simulink model "float_sch_TemplateMatchingContinuous"  (R2020a)
settings: Solver=VariableStepAuto  StartTime=0  StopTime=5  RelTol=1e-3
values from neighbouring files (symbols this model uses):
  buffer_rec = length(template)    [float_sch_run_TemplateMatchingCentered.m]    (also in float_sch_run_TemplateMatchingContinuous.m)
  fs = 30000    [float_sch_run_TemplateMatchingCentered.m]    (also in float_sch_run_TemplateMatchingContinuous.m)
  refractory = 10^-3    (= 0.001)    [float_sch_run_TemplateMatchingCentered.m]    (also in float_sch_run_TemplateMatchingContinuous.m)
  score = [4500]    [float_sch_run_TemplateMatchingCentered.m]    (also in float_sch_run_TemplateMatchingContinuous.m)
  template = double(mean_waveform{1, 1})'    [float_sch_run_TemplateMatchingCentered.m]    (also in float_sch_run_TemplateMatchingContinuous.m)
libraries: dsparch4 x2, simulink x2, dspswit3 x1, hdlsllib x1
settings Model: Creator=sbuccelli  LastModifiedBy=diflo

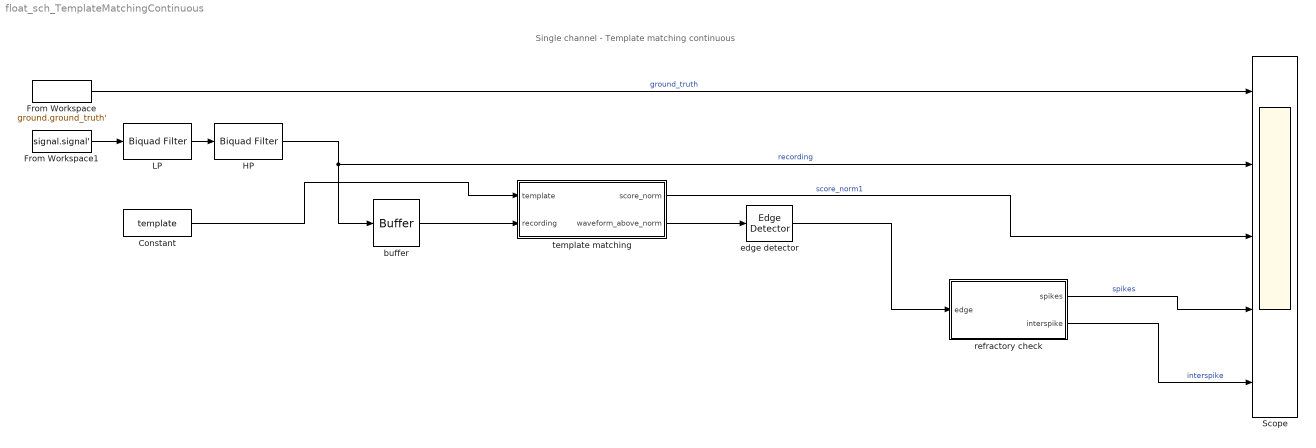
== system float_sch_TemplateMatchingContinuous ==
  note: Single channel - Template matching continuous
  Constant : Constant  Value=template
  From Workspace : FromWorkspace  VariableName=ground.ground_truth'  SampleTime=1/fs
  From Workspace1 : FromWorkspace  VariableName=signal.signal'  SampleTime=1/fs
  HP : dsparch4/Biquad Filter  Tag=BlockMethodSubSystem  FilterSource=Dialog parameters  CoeffSource=Specify via dialog  FilterObject=BQF  IIRFiltStruct=Direct form II  BiQuadCoeffs=[1 -2 1 1 -1.93529438685999167 0.93912079880642374;1 -1 0 1 -0.939062505817492399 0]  ScaleValues=[0.968603796416603768;0.969531252908746199;1]  IC=0  ICnum=0  ICden=0  a0Flag=Warning  optimizeScaleValues=on  ScaleValueMode=Specify via input port (g)  roundingMode=Floor  overflowMode=off  scaleValueFracLength=14  denProdOutputFracLength=30  denAccumFracLength=30  secondMemoryFracLength=15
  LP : dsparch4/Biquad Filter  Tag=BlockMethodSubSystem  FilterSource=Dialog parameters  CoeffSource=Specify via dialog  FilterObject=BQF  IIRFiltStruct=Direct form II  BiQuadCoeffs=[1 1 0 1 -0.509525449494428795 0]  ScaleValues=[0.245237275252785547;1]  IC=0  ICnum=0  ICden=0  a0Flag=Warning  optimizeScaleValues=on  ScaleValueMode=Specify via input port (g)  roundingMode=Floor  overflowMode=off  scaleValueFracLength=14  denProdOutputFracLength=30  denAccumFracLength=30  secondMemoryFracLength=15
  Scope : Scope  NumInputPorts=5
  buffer : Buffer  N=buffer_rec  V=buffer_overlap  OutputFrames=off
  edge detector : dspswit3/Edge Detector  InputProcessing=Columns as channels (frame based)
      settings: SourceProductBaseCode=DS
  refractory check : Subsystem
  template matching : Subsystem
  wires:
  Constant/1 -> template matching/1(template)
  HP/1 -> Scope/2, buffer/1  "recording"
  buffer/1 -> template matching/2(recording)
  From Workspace1/1 -> LP/1
  template matching/2(waveform_above_norm) -> edge detector/1
  From Workspace/1 -> Scope/1  "ground_truth"
  template matching/1(score_norm) -> Scope/3  "score_norm1"
  edge detector/1 -> refractory check/1("  edge")
  refractory check/1(" spikes") -> Scope/4  "spikes"
  refractory check/2(interspike) -> Scope/5  "interspike"
  LP/1 -> HP/1

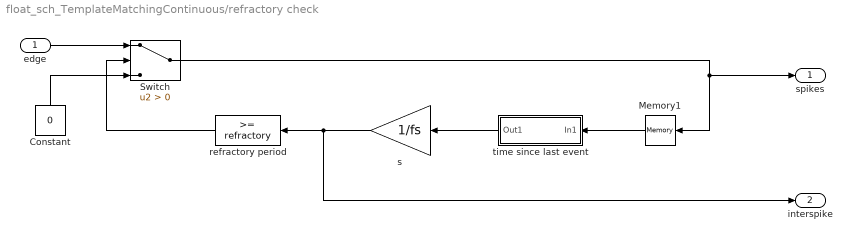
== system float_sch_TemplateMatchingContinuous/refractory check ==
  "  edge" : Inport
  Constant : Constant  Value=0
  Memory1 : Memory  InheritSampleTime=on
  Switch : Switch  Criteria=u2 > Threshold
  refractory period : simulink/Logic and Bit Operations/Compare To Constant  relop=>=  const=refractory  OutDataTypeStr=boolean
  s : Gain  Gain=1/fs  ParamDataTypeStr=double
  time since last event : Subsystem
  " spikes" : Outport
  interspike : Outport  Port=2
  wires:
  "  edge"/1 -> Switch/1
  Memory1/1 -> time since last event/1(In1)
  time since last event/1(Out1) -> s/1
  Constant/1 -> Switch/3
  s/1 -> refractory period/1, interspike/1
  Switch/1 -> " spikes"/1, Memory1/1
  refractory period/1 -> Switch/2

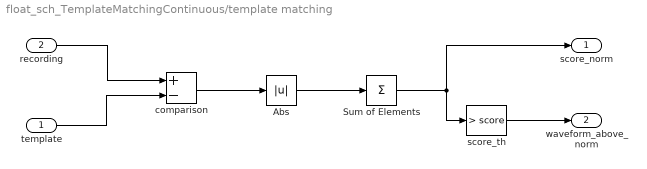
== system float_sch_TemplateMatchingContinuous/template matching ==
  template : Inport
  recording : Inport  Port=2
  Abs : Abs
  Sum of Elements : Sum  Inputs=+
  comparison : Sum  Inputs=+-
  score_th : simulink/Logic and Bit Operations/Compare To Constant  relop=>  const=score  OutDataTypeStr=boolean
  score_norm : Outport
  waveform_above_norm : Outport  Port=2
  wires:
  Abs/1 -> Sum of Elements/1
  comparison/1 -> Abs/1
  Sum of Elements/1 -> score_th/1, score_norm/1
  recording/1 -> comparison/1
  score_th/1 -> waveform_above_norm/1
  template/1 -> comparison/2

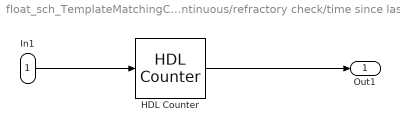
== system float_sch_TemplateMatchingContinuous/refractory check/time since last event ==
  In1 : Inport
  HDL Counter : hdlsllib/Sources/HDL Counter  CountType=Free running  CountInit=1  CountStep=1  CountMax=25  CountFromType=Initial value  CountFrom=1  CountResetPort=on  CountLoadPort=off  CountEnbPort=off  CountDirPort=off  CountDataType=Unsigned  CountWordLen=32  CountFracLen=0  CountSampTime=1
  Out1 : Outport
  wires:
  In1/1 -> HDL Counter/1
  HDL Counter/1 -> Out1/1
